simulink model "VFrigoureuse_fonctionneMal"  (R2021b)
settings: Solver=ode15s  StartTime=0.0  StopTime=1500  RelTol=1e-3
settings Model: Creator=elina  LastModifiedBy=elina

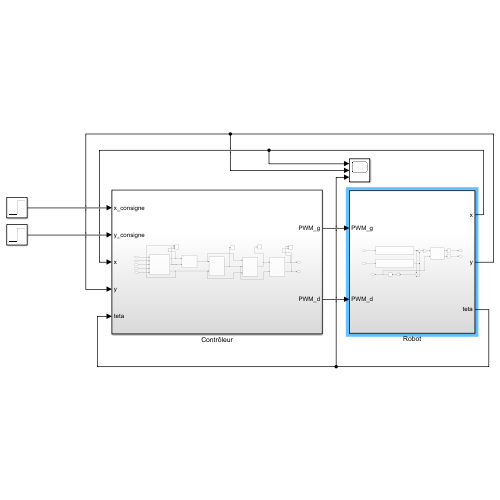
[thumbnail: Simulink's stored preview of the top-level diagram]
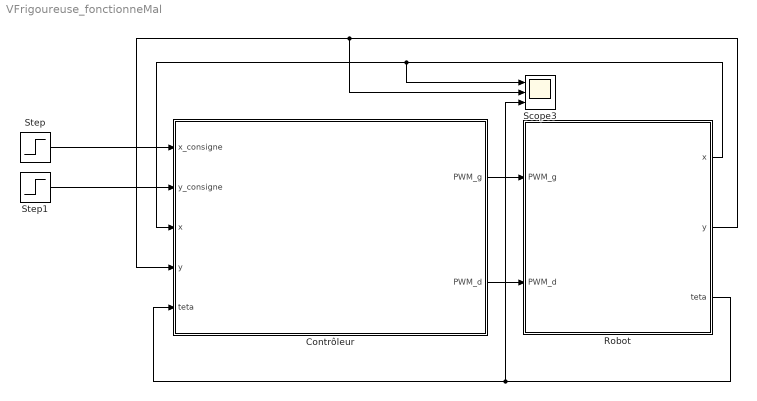
== system VFrigoureuse_fonctionneMal ==
  Contrôleur : Subsystem
  Robot : Subsystem
  Scope3 : Scope  NumInputPorts=3
  Step : Step  Time=0  After=10  SampleTime=0
  Step1 : Step  Time=0  After=10  SampleTime=0
  wires:
  Robot/1(x) -> Scope3/1, Contrôleur/3(x)
  Robot/2(y) -> Scope3/2, Contrôleur/4(y)
  Step/1 -> Contrôleur/1(x_consigne)
  Step1/1 -> Contrôleur/2(y_consigne)
  Contrôleur/1(PWM_g) -> Robot/1(PWM_g)
  Contrôleur/2(PWM_d) -> Robot/2(PWM_d)
  Robot/3(teta) -> Scope3/3, Contrôleur/5(teta)

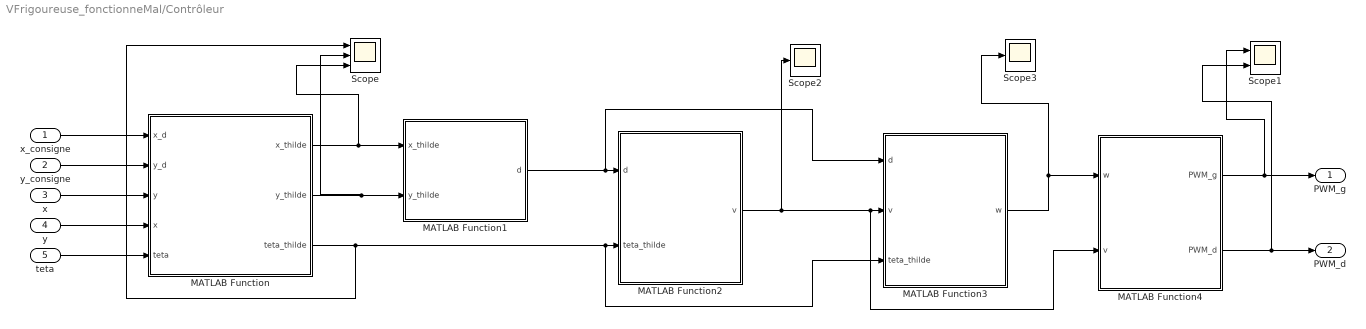
== system VFrigoureuse_fonctionneMal/Contrôleur ==
  x_consigne : Inport
  y_consigne : Inport  Port=2
  x : Inport  Port=3
  y : Inport  Port=4
  teta : Inport  Port=5
  MATLAB Function : MATLAB Function  TreatAsAtomicUnit=on
  MATLAB Function1 : MATLAB Function  TreatAsAtomicUnit=on
  MATLAB Function2 : MATLAB Function  TreatAsAtomicUnit=on
  MATLAB Function3 : MATLAB Function  TreatAsAtomicUnit=on
  MATLAB Function4 : MATLAB Function  TreatAsAtomicUnit=on
  Scope : Scope  NumInputPorts=3
  Scope1 : Scope  NumInputPorts=2
  Scope2 : Scope
  Scope3 : Scope
  PWM_g : Outport
  PWM_d : Outport  Port=2
  wires:
  y/1 -> MATLAB Function/4(x)
  MATLAB Function4/2(PWM_d) -> Scope1/2, PWM_d/1
  MATLAB Function/1(x_thilde) -> Scope/3, MATLAB Function1/1(x_thilde)
  MATLAB Function2/1(v) -> Scope2/1, MATLAB Function4/2(v), MATLAB Function3/2(v)
  MATLAB Function3/1(w) -> Scope3/1, MATLAB Function4/1(w)
  y_consigne/1 -> MATLAB Function/2(y_d)
  x/1 -> MATLAB Function/3(y)
  teta/1 -> MATLAB Function/5(teta)
  MATLAB Function1/1(d) -> MATLAB Function3/1(d), MATLAB Function2/1(d)
  MATLAB Function/2(y_thilde) -> Scope/2, MATLAB Function1/2(y_thilde)
  x_consigne/1 -> MATLAB Function/1(x_d)
  MATLAB Function/3(teta_thilde) -> Scope/1, MATLAB Function3/3(teta_thilde), MATLAB Function2/2(teta_thilde)
  MATLAB Function4/1(PWM_g) -> Scope1/1, PWM_g/1

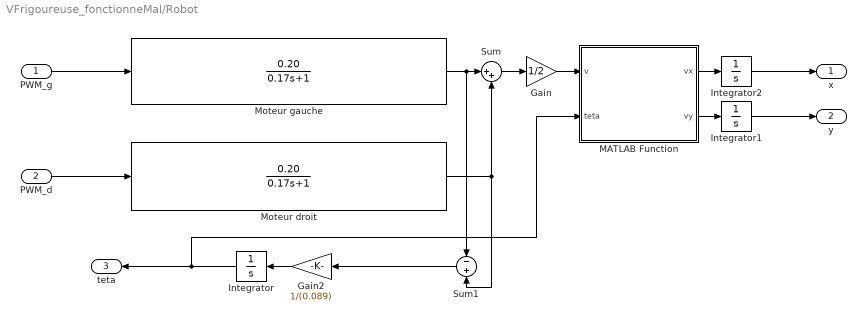
== system VFrigoureuse_fonctionneMal/Robot ==
  PWM_g : Inport
  PWM_d : Inport  Port=2
  Gain : Gain  Gain=1/2
  Gain2 : Gain  Gain=1/(0.089)
  Integrator : Integrator
  Integrator1 : Integrator
  Integrator2 : Integrator
  MATLAB Function : MATLAB Function  TreatAsAtomicUnit=on
  Moteur droit : TransferFcn  Numerator=[0.20]  Denominator=[0.17 1 ]
  Moteur gauche : TransferFcn  Numerator=[0.20]  Denominator=[0.17 1 ]
  Sum : Sum  Inputs=|++
  Sum1 : Sum  Inputs=-+
  x : Outport
  y : Outport  Port=2
  teta : Outport  Port=3
  wires:
  Integrator/1 -> teta/1, MATLAB Function/2(teta)
  Gain2/1 -> Integrator/1
  MATLAB Function/2(vy) -> Integrator1/1
  Moteur gauche/1 -> Sum/1, Sum1/1
  Gain/1 -> MATLAB Function/1(v)
  MATLAB Function/1(vx) -> Integrator2/1
  Moteur droit/1 -> Sum1/2, Sum/2
  Sum/1 -> Gain/1
  Sum1/1 -> Gain2/1
  PWM_d/1 -> Moteur droit/1
  PWM_g/1 -> Moteur gauche/1
  Integrator1/1 -> y/1
  Integrator2/1 -> x/1

== matlab function VFrigoureuse_fonctionneMal/Contrôleur/MATLAB Function1 ==
  data: x_thilde input; d output; y_thilde input
function d =distance(x_thilde,y_thilde)
d=(x_thilde*x_thilde+y_thilde*y_thilde)^(1/2);
end

== matlab function VFrigoureuse_fonctionneMal/Contrôleur/MATLAB Function ==
  data: x_d input; x_thilde output; y_d input; y input; x input; teta input; y_thilde output; teta_thilde output
function [x_thilde,y_thilde,teta_thilde]=thilde(x_d,y_d,y,x,teta)
x_thilde=x_d-x;
y_thilde=y_d-y;
%teta=atan2(sin(teta),cos(teta));
teta_thilde=atan2(y_thilde,x_thilde)-teta;
if teta_thilde>pi
    teta_thilde=teta_thilde-2*pi;
elseif teta_thilde<-pi
    teta_thilde=teta_thilde+2*pi;
end
%teta_thilde=atan2(y_thilde,x_thilde);
end

== matlab function VFrigoureuse_fonctionneMal/Contrôleur/MATLAB Function2 ==
  data: d input; v output; teta_thilde input
function v  =vitesse(d,teta_thilde)
k1=0.5;
k3=2;
v_max=0.32;
v=abs((d/(k1+d))*v_max*cos(k3*teta_thilde));
end

== matlab function VFrigoureuse_fonctionneMal/Contrôleur/MATLAB Function3 ==
  data: d input; v input; w output; teta_thilde input
function w  =vitesse_angulaire(d,v,teta_thilde)
k2=1;
k3=1;
if d<0.01
    w=(v/0.01)*sin(teta_thilde)+k2*tanh(k3*teta_thilde);

else
    w=(v/d)*sin(teta_thilde)+k2*tanh(k3*teta_thilde);
end
end

== matlab function VFrigoureuse_fonctionneMal/Contrôleur/MATLAB Function4 ==
  data: w input; v input; PWM_g output; PWM_d output
function [PWM_g,PWM_d]  =consignes(w,v)
delta=0.089;
Ks=0.20;
M=[-1/delta 1/delta;1/2 1/2];
P=inv(M);
V=P*[w;v];
v_g=V(1);
v_d=V(2);
PWM_g=v_g/Ks;
PWM_d=v_d/Ks;
end

== matlab function VFrigoureuse_fonctionneMal/Robot/MATLAB Function ==
  data: v input; teta input; vx output; vy output
function [vx,vy] = vitesse_lineaire(v,teta)
vx=v*cos(teta);
vy=v*sin(teta);
end
